simulink model "ultimointento"  (Simulink 7.9)
settings: Solver=ode45  StartTime=0.0  StopTime=50  RelTol=1e-3
settings Model: Creator=Miguel Faggioni  LastModifiedBy=Miguel Faggioni
settings DataIOCC: TimeSaveName=t  OutputSaveName=y

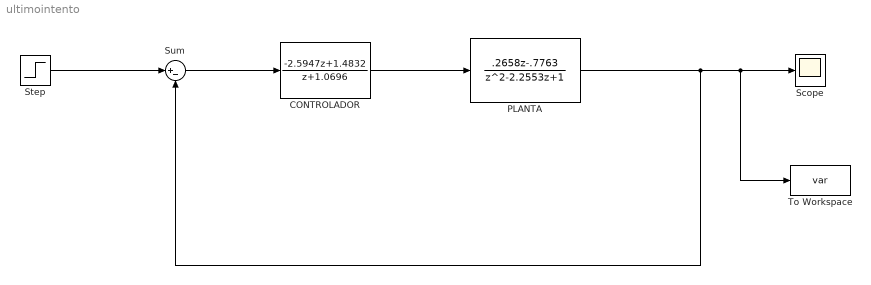
== system ultimointento ==
  CONTROLADOR : DiscreteTransferFcn  Numerator=[-2.5947 1.4832]  Denominator=[1 1.0696]
  PLANTA : DiscreteTransferFcn  Numerator=[.2658 -.7763]  Denominator=[1 -2.2553 1]
  Scope : Scope
  Step : Step  Time=0  SampleTime=.05
  Sum : Sum  Inputs=|+-
  To Workspace : ToWorkspace  VariableName=var  SampleTime=-1
  wires:
  Sum/1 -> CONTROLADOR/1
  CONTROLADOR/1 -> PLANTA/1
  PLANTA/1 -> Sum/2, Scope/1, To Workspace/1
  Step/1 -> Sum/1
